simulink model "main_sim_adapt_Gref_SPPH"  (Simulink 7.2)
settings: Solver=ode2  SolverMode=SingleTasking  StartTime=0.0  StopTime=tsim_max  FixedStep=dtsim  RelTol=1e-3
StopFcn:
  | %mkplt
values from neighbouring files (symbols this model uses):
  assertion_time = inf    [setup_taem_sgs_al.m]
  cosA = cos(rwyAZ_rad)    [setup_taem_sgs_al.m]
  E_rwy = E_origin + (mod(( rwyLLA(2)/constants.r2d - lon_origin )+pi,2*pi)-pi) * constants.earth_radius * cos(lat_origin)    [setup_taem_sgs_al.m]
  eow_boundary = tmp_eow(ix(1))    [setup_taem_sgs_al.m]
  N_rwy = N_origin + (mod(( rwyLLA(1)/constants.r2d - lat_origin )+pi,2*pi)-pi) * constants.earth_radius    [setup_taem_sgs_al.m]
  sinA = sin(rwyAZ_rad)    [setup_taem_sgs_al.m]
  vel = 487.2512    [doit.m]
undefined symbols (not defined in the file or in its folder): accel_cmd, aero_surf_qbar_off, aero_surf_qbar_on, Alon, att_cmd_select, att_trim_IC, att_type, att_type_numbers, B1, bb_ellipsoid, bb_params, Blon, C, CA, chi_trim_IC, Clon, command_time, compute_all_rate_cols, compute_all_vel_cols, constants, da_trim_IC, dc_L2W_IC, de_trim_IC, DiscIntNeverNeededParam, dr_trim_IC, dtsim, DZkx, DZtheta, E_trim_IC, Ed_cmd, Ed_trim_IC, fc, flag_uad, full_surf_llim, full_surf_ulim, gain_set, gain_var_struct, gam_cmd_descent, gam_cmd_preflare, gamdot_cmd_descent, gamdot_cmd_flare, gamdot_cmd_preflare, gamma_trim_IC, Gamtheta, Gamx, h_trim_IC, hd_cmd, hd_trim_IC, ideal_vel_Kb, in_exsig_vecin, in_exsig_vecout, invCB, Kb, Kxhat0, Kxnom, Kxstar, lonxm0, MACH, MACH_att_fb, MACH_att_int_IC ... (+77)
libraries: simulink x36, utility_lib x36, mach_lib x24, model_lib x15, simulink_need_slupdate x8, models x6
(part 1 of 7)
CloseFcn:
  | rtwprivate ssgencode ModelCloseRequest main
settings Model: Creator=E183308  LastModifiedBy=E183308  ModifiedComment=E700252 -- Tue Nov 11 13:33:23 2003 -- Version 1.2477  TunableVars=MACH_U_nom_IC,MACH_gain_mat,MACH_mass_IC,MACH_pos_IC,MACH_pqr_Bmat_IC,MACH_pqr_u_IC,MACH_quat_IC,MACH_throttle_IC,MACH_vel_Bmat_IC,MACH_vel_IC,MACH_vel_cvdnom_IC,MACH_vel_uold_IC  TunableVarsStorageClass=Auto,Auto,Auto,Auto,Auto,Auto,Auto,Auto,Auto,Auto,Auto,Auto  TunableVarsTypeQualifier=,,,,,,,,,,,  BufferReuse=off
settings DataIOCC: LimitDataPoints=off  SaveOutput=off  SaveTime=off  SignalLoggingName=sigsOut
settings OptimizationCC: BlockReduction=off  BooleanDataType=off  BufferReuse=off  EnforceIntegerDowncast=off  FoldNonRolledExpr=off  InitFltsAndDblsToZero=on
settings DebuggingCC: SaveWithParameterizedLinksMsg=none  SignalResolutionControl=TryResolveAllWithWarning  SolverPrmCheckMsg=none  InheritedTsInSrcMsg=none  MultiTaskDSMMsg=warning  MultiTaskCondExecSysMsg=none  StrictBusMsg=ErrorLevel1
settings HardwareCC: TargetEndianess=LittleEndian  TargetHWDeviceType=MATLAB Host  ProdEqTarget=off
settings SFSimCC: SFSimEcho=off
settings RTWCC: SystemTargetFile=rtwsfcn.tlc  TemplateMakefile=rtwsfcn_default_tmf  Description=S-function Target  ProcessScript=rtwsfcn_make_rtw_hook  IncludeERTFirstTime=on
settings STFCustomTargetCC: TargetFcnLib=ansi_tfl_tmw.mat  ModelReferenceCompliant=off  SystemTargetFile=rtwsfcn.tlc
settings CustomProperty: Value=on

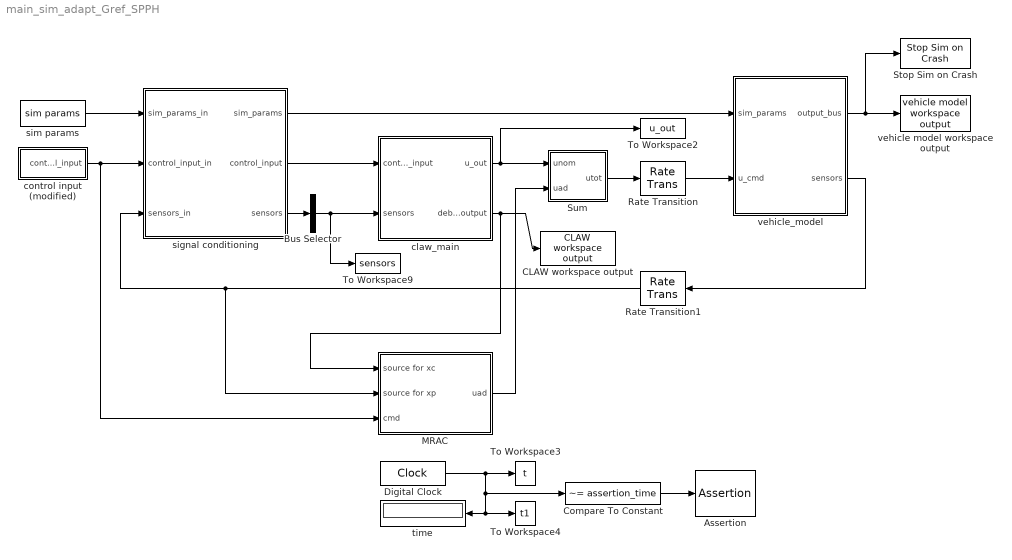
== system main_sim_adapt_Gref_SPPH ==
  Assertion : Assertion  Enabled=on  AssertionFailFcn=assertioncb  StopWhenAssertionFail=off
  Bus Selector : BusSelector  OutputSignals=pqr,NED_dot,latlonh,e,accels_cg,nav_ok,u_meas,NED_wind,seeker  OutputAsBus=on
  CLAW workspace output : mach_lib/CLAW workspace output  SystemSampleTime=-1
  Compare To Constant : simulink/Logic and Bit Operations/Compare To Constant  SystemSampleTime=-1  relop=~=  const=assertion_time  LogicOutDataTypeMode=boolean  ZeroCross=off
  Digital Clock : DigitalClock  SampleTime=dtsim
  MRAC : Subsystem  TreatAsAtomicUnit=on
  Rate Transition : RateTransition  X0=MACH_U_nom_IC
  Rate Transition1 : RateTransition  Orientation=left  OutPortSampleTime=MACH.dt
  Stop Sim on Crash : mach_lib/Stop Sim on Crash  SystemSampleTime=-1
  Sum : Subsystem
  To Workspace2 : ToWorkspace  VariableName=u_out  SampleTime=MACH.dt  SaveFormat=Array
  To Workspace3 : ToWorkspace  VariableName=t  SampleTime=dtsim  SaveFormat=Array
  To Workspace4 : ToWorkspace  VariableName=t1  SampleTime=MACH.dt  SaveFormat=Array
  To Workspace9 : ToWorkspace  VariableName=sensors  SampleTime=MACH.dt  SaveFormat=Array
      settings: MaxDataPoints=1
  claw_main : Subsystem  AncestorBlock=mach_lib/claw_main  TreatAsAtomicUnit=on  SystemSampleTime=MACH.dt
  control input (modified) : Subsystem
  signal conditioning : Subsystem
  sim params : mach_lib/sim params  SystemSampleTime=-1
  time : Display
  vehicle model workspace output : mach_lib/vehicle model workspace output  SystemSampleTime=-1
  vehicle_model : Subsystem  TreatAsAtomicUnit=on
  wires:
  Digital Clock/1 -> To Workspace3/1, Compare To Constant/1, time/1, To Workspace4/1
  claw_main/1(u_out) -> Sum/1(unom), To Workspace2/1
  vehicle_model/2(sensors) -> Rate Transition1/1
  claw_main/2(debug_output) -> CLAW workspace output/1, MRAC/1(source for xc)
  Rate Transition/1 -> vehicle_model/2(u_cmd)
  Bus Selector/1 -> To Workspace9/1, claw_main/2(sensors)
  vehicle_model/1(output_bus) -> vehicle model workspace output/1, Stop Sim on Crash/1
  Rate Transition1/1 -> signal conditioning/3(sensors_in), MRAC/2(source for xp)
  signal conditioning/3(sensors) -> Bus Selector/1
  signal conditioning/2(control_input) -> claw_main/1(control_input)
  sim params/1 -> signal conditioning/1(sim_params_in)
  signal conditioning/1(sim_params) -> vehicle_model/1(sim_params)
  Compare To Constant/1 -> Assertion/1
  MRAC/1(uad) -> Sum/2(uad)
  Sum/1(utot) -> Rate Transition/1
  control input (modified)/1(control_input) -> signal conditioning/2(control_input_in), MRAC/3(cmd)

== system main_sim_adapt_Gref_SPPH/MRAC ==
  source for xc : Inport
  source for xp : Inport  Port=2
  cmd : Inport  Port=3
  Adapt on (1.0 to 15 sec) : Subsystem  Tag=STV Subsys  LoadFcn=sigbuilder_block('load');  StartFcn=sigbuilder_block('start');  StopFcn=sigbuilder_block('stop');  ClipboardFcn=sigbuilder_block('clipboard');  mask(Sigbuilder block){}
      mask help: Sigbuilder GUI
      mask init:
      | if ~strcmp(get_param(bdroot(gcbh),'SimulationStatus'),'stopped') tuvar = sigbuilder_block('maskInit'); end
      settings: CopyFcn=sigbuilder_block('copy');  DeleteFcn=sigbuilder_block('delete');  ModelCloseFcn=sigbuilder_block('modelClose');  PreSaveFcn=sigbuilder_block('preSave');  NameChangeFcn=sigbuilder_block('namechange');  OpenFcn=sigbuilder_block('open',[223.5 120 685.5 399.75 ]);  CloseFcn=sigbuilder_block('close');
      mask Display: plot(0,0,100,100,[10,10,40,40,10],[80,20,20,80,80],[40,10],[50,50], [40,27,10],[65,72,56],[40,25,25,10],[28,28,43,43]);
  Bus Selector1 : BusSelector  OutputSignals=command  OutputAsBus=on
  Estimate of x : Subsystem
  MRAC Laws : Subsystem
  Ref Model (Short Period + Phugoid) : Subsystem
  Selector : Selector  InputPortWidth=4  IndexOptions=Index vector (dialog)  Indices=[2]  OutputSizes=1
  Sum : Sum  Inputs=-|+  OutDataType=sfix(16)  OutScaling=2^0
  Terminator : Terminator
  Terminator1 : Terminator
  To Workspace1 : ToWorkspace  VariableName=uad_xm  SampleTime=MACH.dt  SaveFormat=Array
  To Workspace2 : ToWorkspace  VariableName=uad_conv  SampleTime=MACH.dt  SaveFormat=Array
  To Workspace3 : ToWorkspace  VariableName=uad_x  SampleTime=MACH.dt  SaveFormat=Array
  command : Scope
      settings: YMin=0  YMax=15  SaveName=ScopeData6
  uad out : Scope
      settings: SaveName=ScopeData15
  uad : Outport  OutDataType=sfix(16)  OutScaling=2^0
  wires:
  Bus Selector1/1 -> Selector/1, MRAC Laws/3(r), command/1
  Selector/1 -> Ref Model (Short Period + Phugoid)/1(cmd)
  cmd/1 -> Bus Selector1/1
  MRAC Laws/1(uad) -> uad out/1, uad/1
  MRAC Laws/3(Kx_hat) -> Terminator/1
  MRAC Laws/4(Theta_hat) -> Terminator1/1
  source for xp/1 -> Estimate of x/2(In2)
  source for xc/1 -> Estimate of x/1(In1)
  Estimate of x/1(x) -> Sum/2, MRAC Laws/2(x), To Workspace3/1
  Sum/1 -> MRAC Laws/1(e)
  Adapt on (1.0 to 15 sec)/1(Signal 1) -> MRAC Laws/4(adapt on-off)
  MRAC Laws/2(uad_conv) -> To Workspace2/1
  Ref Model (Short Period + Phugoid)/1(xm) -> Sum/1, To Workspace1/1

== system main_sim_adapt_Gref_SPPH/Sum ==
  unom : Inport
  uad : Inport  Port=2
  Rate Transition1 : RateTransition  OutPortSampleTime=MACH.dt
  Sum : Sum  Inputs=|++  OutDataType=sfix(16)  OutScaling=2^0
  To Workspace1 : ToWorkspace  VariableName=elev_nom  SampleTime=MACH.dt  SaveFormat=Array
  To Workspace2 : ToWorkspace  VariableName=elev_adap  SampleTime=MACH.dt  SaveFormat=Array
  To Workspace9 : ToWorkspace  VariableName=elev_total  SampleTime=MACH.dt  SaveFormat=Array
  get RIE : Selector  InputPortWidth=MACH.num_u  IndexOptions=Index vector (dialog)  Indices=MACH.u_idx.elev  OutputSizes=1
  set RIE : Assignment  IndexOptions=Index vector (dialog)  Indices=MACH.u_idx.elev  OutputSizes=[1 1]
  utot : Outport
  wires:
  unom/1 -> get RIE/1, set RIE/1
  get RIE/1 -> Sum/1, To Workspace1/1
  uad/1 -> Rate Transition1/1
  Sum/1 -> set RIE/2, To Workspace9/1
  set RIE/1 -> utot/1
  Rate Transition1/1 -> To Workspace2/1, Sum/2

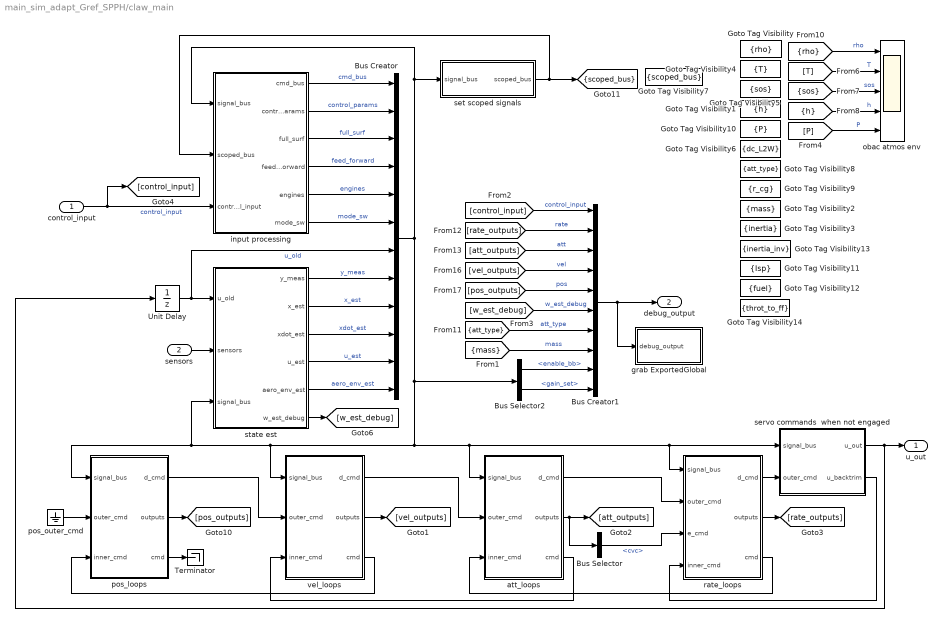
== system main_sim_adapt_Gref_SPPH/claw_main ==
  control_input : Inport  OutDataType=sfix(16)  OutScaling=2^0
      settings: BusObject=control_input_bus
  sensors : Inport  Port=2  OutDataType=sfix(16)  OutScaling=2^0
  Bus Creator : BusCreator  Inputs=12
  Bus Creator1 : BusCreator  Inputs=10
      settings: BusObject=CLAW_DEBUG_OUTPUT_BUS
  Bus Selector : BusSelector  OutputSignals=cvc
  Bus Selector2 : BusSelector  OutputSignals=control_params.enable_bb,control_params.gain_set
  Goto Tag Visibility : GotoTagVisibility  GotoTag=rho
  Goto Tag Visibility1 : GotoTagVisibility  GotoTag=h
  Goto Tag Visibility10 : GotoTagVisibility  GotoTag=P
  Goto Tag Visibility11 : GotoTagVisibility  GotoTag=Isp
  Goto Tag Visibility12 : GotoTagVisibility  GotoTag=fuel
  Goto Tag Visibility13 : GotoTagVisibility  GotoTag=inertia_inv
  Goto Tag Visibility14 : GotoTagVisibility  GotoTag=throt_to_ff
  Goto Tag Visibility2 : GotoTagVisibility  GotoTag=mass
  Goto Tag Visibility3 : GotoTagVisibility  GotoTag=inertia
  Goto Tag Visibility4 : GotoTagVisibility  GotoTag=T
  Goto Tag Visibility5 : GotoTagVisibility  GotoTag=sos
  Goto Tag Visibility6 : GotoTagVisibility  GotoTag=dc_L2W
  Goto Tag Visibility7 : GotoTagVisibility  GotoTag=scoped_bus
  Goto Tag Visibility8 : GotoTagVisibility  GotoTag=att_type
  Goto Tag Visibility9 : GotoTagVisibility  GotoTag=r_cg
  Terminator : Terminator
  Unit Delay : UnitDelay  X0=MACH_U_nom_IC  SampleTime=-1
  att_loops : Subsystem
  grab ExportedGlobal : Subsystem
  input processing : Subsystem
  obac atmos env : Scope  NumInputPorts=5
      settings: YMin=-5~-5~-5~-5~-5  YMax=5~5~5~5~5  SaveName=ScopeData2
  pos_loops : Subsystem
      settings: RTWSystemCode=Function
  pos_outer_cmd : Ground
  rate_loops : Subsystem
      settings: RTWSystemCode=Function
  servo commands  when not engaged : Subsystem
  set scoped signals : Subsystem
  state est : Subsystem
  vel_loops : Subsystem
      settings: RTWSystemCode=Function
  u_out : Outport  OutDataType=sfix(16)  OutScaling=2^0
  debug_output : Outport  Port=2  OutDataType=sfix(16)  OutScaling=2^0
  tag scope: scoped_bus=scoped
  wires:
  input processing/6(mode_sw) -> Bus Creator/6  "mode_sw"
  input processing/5(engines) -> Bus Creator/5  "engines"
  pos_loops/2(outputs) -> [pos_outputs]
  [pos_outputs] -> Bus Creator1/5  "pos"
  [vel_outputs] -> Bus Creator1/4  "vel"
  [att_outputs] -> Bus Creator1/3  "att"
  [rate_outputs] -> Bus Creator1/2  "rate"
  att_loops/1(d_cmd) -> rate_loops/2(outer_cmd)
  vel_loops/1(d_cmd) -> att_loops/2(outer_cmd)
  rate_loops/1(d_cmd) -> servo commands  when not engaged/2(outer_cmd)
  Bus Creator/1 -> att_loops/1(signal_bus), rate_loops/1(signal_bus), servo commands  when not engaged/1(signal_bus), vel_loops/1(signal_bus), pos_loops/1(signal_bus), state est/3(signal_bus), Bus Selector2/1, input processing/1(signal_bus), set scoped signals/1(signal_bus)
  pos_loops/3(cmd) -> Terminator/1
  att_loops/3(cmd) -> vel_loops/3(inner_cmd)
  rate_loops/3(cmd) -> att_loops/3(inner_cmd)
  pos_loops/1(d_cmd) -> vel_loops/2(outer_cmd)
  vel_loops/2(outputs) -> [vel_outputs]
  att_loops/2(outputs) -> [att_outputs], Bus Selector/1
  rate_loops/2(outputs) -> [rate_outputs]
  Bus Creator1/1 -> debug_output/1, grab ExportedGlobal/1(debug_output)
  Unit Delay/1 -> state est/1(u_old), Bus Creator/7  "u_old"
  sensors/1 -> state est/2(sensors)
  vel_loops/3(cmd) -> pos_loops/3(inner_cmd)
  servo commands  when not engaged/2(u_backtrim) -> rate_loops/4(inner_cmd)
  state est/4(u_est) -> Bus Creator/11  "u_est"
  state est/3(xdot_est) -> Bus Creator/10  "xdot_est"
  state est/2(x_est) -> Bus Creator/9  "x_est"
  state est/1(y_meas) -> Bus Creator/8  "y_meas"
  servo commands  when not engaged/1(u_out) -> u_out/1, Unit Delay/1
  pos_outer_cmd/1 -> pos_loops/2(outer_cmd)
  state est/6(w_est_debug) -> [w_est_debug]
  [w_est_debug] -> Bus Creator1/6  "w_est_debug"
  [att_type] -> Bus Creator1/7  "att_type"
  input processing/2(control_params) -> Bus Creator/2  "control_params"
  [h] -> obac atmos env/4  "h"
  [sos] -> obac atmos env/3  "sos"
  [T] -> obac atmos env/2  "T"
  [rho] -> obac atmos env/1  "rho"
  [P] -> obac atmos env/5  "P"
  state est/5(aero_env_est) -> Bus Creator/12  "aero_env_est"
  input processing/3(full_surf) -> Bus Creator/3  "full_surf"
  input processing/4(feed_forward) -> Bus Creator/4  "feed_forward"
  set scoped signals/1(scoped_bus) -> [scoped_bus], input processing/2(scoped_bus)
  [mass] -> Bus Creator1/8  "mass"
  Bus Selector2/1 -> Bus Creator1/9  "<enable_bb>"
  Bus Selector2/2 -> Bus Creator1/10  "<gain_set>"
  control_input/1 -> input processing/3(control_input), [control_input]  "control_input"
  input processing/1(cmd_bus) -> Bus Creator/1  "cmd_bus"
  [control_input] -> Bus Creator1/1  "control_input"
  Bus Selector/1 -> rate_loops/3(e_cmd)  "<cvc>"

== system main_sim_adapt_Gref_SPPH/control input (modified) ==
  Add Excitation : Subsystem
  Bus Assignment : BusAssignment  AssignedSignals=command
  control input : Subsystem  AncestorBlock=mach_lib/control input  SystemSampleTime=MACH.dt
  ideal responses : Subsystem  AncestorBlock=model_lib/ideal responses
  control_input : Outport
  wires:
  control input/1(control_input) -> Bus Assignment/1, Add Excitation/1(In)
  Add Excitation/1(Out) -> Bus Assignment/2
  Bus Assignment/1 -> control_input/1, ideal responses/1(control_input)

== system main_sim_adapt_Gref_SPPH/signal conditioning ==
  sim_params_in : Inport  OutDataType=sfix(16)  OutScaling=2^0
  control_input_in : Inport  Port=2  OutDataType=sfix(16)  OutScaling=2^0
  sensors_in : Inport  Port=3  OutDataType=sfix(16)  OutScaling=2^0
  Bus Assignment : BusAssignment  AssignedSignals=full_surf.full_surf_pref
  Bus Selector : BusSelector  OutputSignals=full_surf.full_surf_pref
  Compare To Constant : simulink/Logic and Bit Operations/Compare To Constant  SystemSampleTime=-1  relop=>=  const=0  LogicOutDataTypeMode=boolean  ZeroCross=off
  Compare To Constant1 : simulink/Logic and Bit Operations/Compare To Constant  SystemSampleTime=-1  relop=<=  const=5  LogicOutDataTypeMode=boolean  ZeroCross=off
  Constant : Constant  Value=360  OutDataType=sfix(16)  OutScaling=2^0
  Digital Clock : DigitalClock  SampleTime=MACH.dt
  Gain : Gain  Gain=0  ParameterDataType=sfix(16)  ParameterScaling=2^0  OutDataType=sfix(16)  OutScaling=2^0
  Logical Operator : Logic  AllPortsSameDT=off
  Product : Product  OutDataType=sfix(16)  OutScaling=2^0  RndMeth=Zero
  Sine Wave : Sin  TimeSource=Use external signal  Amplitude=5  Frequency=2*pi  SampleTime=0
  Sum : Sum  Inputs=|++  OutDataType=sfix(16)  OutScaling=2^0
  Sum1 : Sum  Inputs=|+-  OutDataType=sfix(16)  OutScaling=2^0
  get RIE : Selector  InputPortWidth=MACH.num_u  IndexOptions=Index vector (dialog)  Indices=MACH.vane_idx(1)  OutputSizes=1
  set RIE : Assignment  IndexOptions=Index vector (dialog)  Indices=MACH.vane_idx(1)  OutputSizes=[1 1]
  sim_params : Outport  OutDataType=sfix(16)  OutScaling=2^0
  control_input : Outport  Port=2  OutDataType=sfix(16)  OutScaling=2^0
  sensors : Outport  Port=3  OutDataType=sfix(16)  OutScaling=2^0
  wires:
  sim_params_in/1 -> sim_params/1
  control_input_in/1 -> Bus Assignment/1, Bus Selector/1
  sensors_in/1 -> sensors/1
  set RIE/1 -> Bus Assignment/2
  Sum/1 -> set RIE/2
  Bus Selector/1 -> set RIE/1, get RIE/1  "<full_surf_pref>"
  get RIE/1 -> Sum/1
  Digital Clock/1 -> Sum1/1
  Constant/1 -> Sum1/2
  Sum1/1 -> Sine Wave/1, Compare To Constant/1, Compare To Constant1/1
  Compare To Constant/1 -> Logical Operator/1
  Compare To Constant1/1 -> Logical Operator/2
  Logical Operator/1 -> Product/2
  Sine Wave/1 -> Product/1
  Product/1 -> Gain/1
  Bus Assignment/1 -> control_input/1
  Gain/1 -> Sum/2

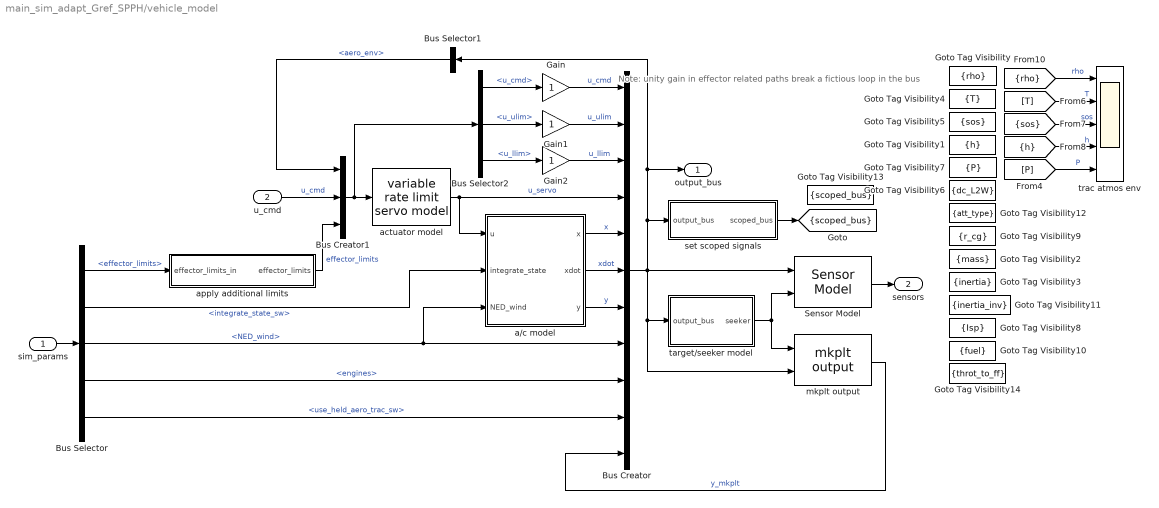
== system main_sim_adapt_Gref_SPPH/vehicle_model ==
  note: Note: unity gain in effector related paths
      | break a fictious loop in the bus
  sim_params : Inport  OutDataType=sfix(16)  OutScaling=2^0
  u_cmd : Inport  Port=2  OutDataType=sfix(16)  OutScaling=2^0
  Bus Creator : BusCreator  Inputs=11
  Bus Creator1 : BusCreator  Inputs=3
  Bus Selector : BusSelector  OutputSignals=effector_limits,integrate_state_sw,NED_wind,engines,use_held_aero_trac_sw
  Bus Selector1 : BusSelector  Orientation=left  OutputSignals=y.aero_env
  Bus Selector2 : BusSelector  OutputSignals=u_cmd,effector_limits.u_ulim,effector_limits.u_llim
  Gain : Gain  ParameterDataType=sfix(16)  ParameterScaling=2^0  OutDataType=sfix(16)  OutScaling=2^0
  Gain1 : Gain  ParameterDataType=sfix(16)  ParameterScaling=2^0  OutDataType=sfix(16)  OutScaling=2^0
  Gain2 : Gain  ParameterDataType=sfix(16)  ParameterScaling=2^0  OutDataType=sfix(16)  OutScaling=2^0
  Goto Tag Visibility : GotoTagVisibility  GotoTag=rho
  Goto Tag Visibility1 : GotoTagVisibility  GotoTag=h
  Goto Tag Visibility10 : GotoTagVisibility  GotoTag=fuel
  Goto Tag Visibility11 : GotoTagVisibility  GotoTag=inertia_inv
  Goto Tag Visibility12 : GotoTagVisibility  GotoTag=att_type
  Goto Tag Visibility13 : GotoTagVisibility  GotoTag=scoped_bus
  Goto Tag Visibility14 : GotoTagVisibility  GotoTag=throt_to_ff
  Goto Tag Visibility2 : GotoTagVisibility  GotoTag=mass
  Goto Tag Visibility3 : GotoTagVisibility  GotoTag=inertia
  Goto Tag Visibility4 : GotoTagVisibility  GotoTag=T
  Goto Tag Visibility5 : GotoTagVisibility  GotoTag=sos
  Goto Tag Visibility6 : GotoTagVisibility  GotoTag=dc_L2W
  Goto Tag Visibility7 : GotoTagVisibility  GotoTag=P
  Goto Tag Visibility8 : GotoTagVisibility  GotoTag=Isp
  Goto Tag Visibility9 : GotoTagVisibility  GotoTag=r_cg
  Sensor Model : model_lib/Sensor Model  SystemSampleTime=-1
  a/c model : Subsystem
  actuator model : model_lib/variable rate limit servo model  SystemSampleTime=-1
  apply additional limits : Subsystem
  mkplt output : model_lib/mkplt output  SystemSampleTime=-1
  set scoped signals : Subsystem
  target/seeker model : Subsystem
  trac atmos env : Scope  NumInputPorts=5
      settings: YMin=-5~-5~-5~-5~-5  YMax=5~5~5~5~5
  output_bus : Outport  OutDataType=sfix(16)  OutScaling=2^0
  sensors : Outport  Port=2  OutDataType=sfix(16)  OutScaling=2^0
  tag scope: scoped_bus=scoped
  wires:
  actuator model/1 -> a/c model/1(u), Bus Creator/4  "u_servo"
  Sensor Model/1 -> sensors/1
  Bus Selector/3 -> Bus Creator/8, a/c model/3(NED_wind)  "<NED_wind>"
  [h] -> trac atmos env/4  "h"
  [sos] -> trac atmos env/3  "sos"
  [T] -> trac atmos env/2  "T"
  [rho] -> trac atmos env/1  "rho"
  [P] -> trac atmos env/5  "P"
  target/seeker model/1(seeker) -> Sensor Model/2, mkplt output/1
  a/c model/1(x) -> Bus Creator/5  "x"
  a/c model/2(xdot) -> Bus Creator/6  "xdot"
  a/c model/3(y) -> Bus Creator/7  "y"
  Bus Creator/1 -> set scoped signals/1(output_bus), output_bus/1, Bus Selector1/1, target/seeker model/1(output_bus), mkplt output/2, Sensor Model/1
  sim_params/1 -> Bus Selector/1
  set scoped signals/1(scoped_bus) -> [scoped_bus]
  Bus Selector/4 -> Bus Creator/9  "<engines>"
  mkplt output/1 -> Bus Creator/11  "y_mkplt"
  Bus Selector/5 -> Bus Creator/10  "<use_held_aero_trac_sw>"
  Bus Creator1/1 -> actuator model/1, Bus Selector2/1
  Bus Selector1/1 -> Bus Creator1/1  "<aero_env>"
  u_cmd/1 -> Bus Creator1/2  "u_cmd"
  Bus Selector2/1 -> Gain/1  "<u_cmd>"
  Bus Selector2/2 -> Gain1/1  "<u_ulim>"
  Bus Selector2/3 -> Gain2/1  "<u_llim>"
  Gain/1 -> Bus Creator/1  "u_cmd"
  Gain1/1 -> Bus Creator/2  "u_ulim"
  Gain2/1 -> Bus Creator/3  "u_llim"
  Bus Selector/2 -> a/c model/2(integrate_state)  "<integrate_state_sw>"
  Bus Selector/1 -> apply additional limits/1(effector_limits_in)  "<effector_limits>"
  apply additional limits/1(effector_limits) -> Bus Creator1/3  "effector_limits"

== system main_sim_adapt_Gref_SPPH/MRAC/Adapt on (1.0 to 15 sec) ==
  Demux : Demux  Tag=STV Demux  Outputs=1
  FromWs : FromWorkspace  Tag=STV FromWs  VariableName=tuvar  SampleTime=0  SigBuilderData=DataTag0  VnvData=DataTag1
      SigBuilderData=|
      | common.afterFinalStr = 'Extrapolate'
      | common.sampleTime = 0
      | dataSet.timeRange = [0 25]
      | dataSet.name = 'Group 1'
      | sbobj.Groups.Signals.XData = [0 1 1 15 15 25]
      | sbobj.Groups.Signals.YData = [0 0 1 1 0 0]
  Signal 1 : Outport  Tag=STV Outport  OutDataType=sfix(16)  OutScaling=2^0
  wires:
  Demux/1 -> Signal 1/1
  FromWs/1 -> Demux/1

== system main_sim_adapt_Gref_SPPH/MRAC/Estimate of x ==
  In1 : Inport
  In2 : Inport  Port=2
  Bus Selector : BusSelector  OutputSignals=pqr,e,NED_dot,NED_wind
  Bus Selector22 : BusSelector  OutputSignals=rate.integ
  Constant1 : Constant  Orientation=left  Value=4.64*pi/180  OutDataType=sfix(16)  OutScaling=2^0
  Gain3 : Gain  Gain=180/pi  ParameterDataType=sfix(16)  ParameterScaling=2^0  OutDataType=sfix(16)  OutScaling=2^0
  Gain4 : Gain  Gain=180/pi  ParameterDataType=sfix(16)  ParameterScaling=2^0  OutDataType=sfix(16)  OutScaling=2^0
  Gain6 : Gain  Gain=180/pi  ParameterDataType=sfix(16)  ParameterScaling=2^0  OutDataType=sfix(16)  OutScaling=2^0
  K3 : Gain  Gain=-1/(fi*Kb)  ParameterDataType=sfix(16)  ParameterScaling=2^0  OutDataType=sfix(16)  OutScaling=2^0
  Mux : Mux  Inputs=3
  Product : Product  Multiplication=Matrix(*)  OutDataType=sfix(16)  OutScaling=2^0  SaturateOnIntegerOverflow=on  OutDataTypeStr=Inherit: Same as first input
  Reshape : Reshape  OutputDimensionality=Customize  OutputDimensions=[3,3]
  Selector1 : Selector  InputPortWidth=3  IndexOptions=Index vector (dialog)  Indices=[2]  OutputSizes=1
  Selector2 : Selector  InputPortWidth=3  IndexOptions=Index vector (dialog)  Indices=[2]  OutputSizes=1
  Sum1 : Sum  Inputs=|++  OutDataType=sfix(16)  OutScaling=2^0  SaturateOnIntegerOverflow=on
  Sum2 : Sum  Orientation=left  Inputs=|-+  OutDataType=sfix(16)  OutScaling=2^0
  Terminator2 : Terminator
  Terminator3 : Terminator
  alpha : Scope
      settings: YMin=-1  YMax=1  SaveName=ScopeData16
  del alpha : Scope
      settings: YMin=-1  YMax=1  SaveName=ScopeData25
  e2dc : utility_lib/e2dc  SystemSampleTime=-1
  q : Scope
      settings: SaveName=ScopeData11
  uvw_rw2Vab : utility_lib/uvw_rw2Vab  SystemSampleTime=-1
  xc : Scope
      settings: SaveName=ScopeData10
  x : Outport
  wires:
  Bus Selector/1 -> Selector1/1  "<pqr>"
  Bus Selector/2 -> e2dc/1  "<e>"
  Bus Selector22/1 -> Selector2/1  "<integ>"
  Selector2/1 -> K3/1
  e2dc/1 -> Reshape/1
  uvw_rw2Vab/2 -> Gain6/1, Sum2/2  "alpha"
  Gain6/1 -> alpha/1
  Sum1/1 -> Product/2
  Bus Selector/3 -> Sum1/1  "<NED_dot>"
  Bus Selector/4 -> Sum1/2  "<NED_wind>"
  Product/1 -> uvw_rw2Vab/1
  Reshape/1 -> Product/1
  uvw_rw2Vab/1 -> Terminator2/1
  uvw_rw2Vab/3 -> Terminator3/1
  Gain3/1 -> q/1
  Selector1/1 -> Gain3/1, Mux/2  "q"
  Sum2/1 -> Mux/3, Gain4/1
  Constant1/1 -> Sum2/1
  Gain4/1 -> del alpha/1
  In1/1 -> Bus Selector22/1
  Mux/1 -> x/1
  In2/1 -> Bus Selector/1
  K3/1 -> xc/1, Mux/1  "xc"

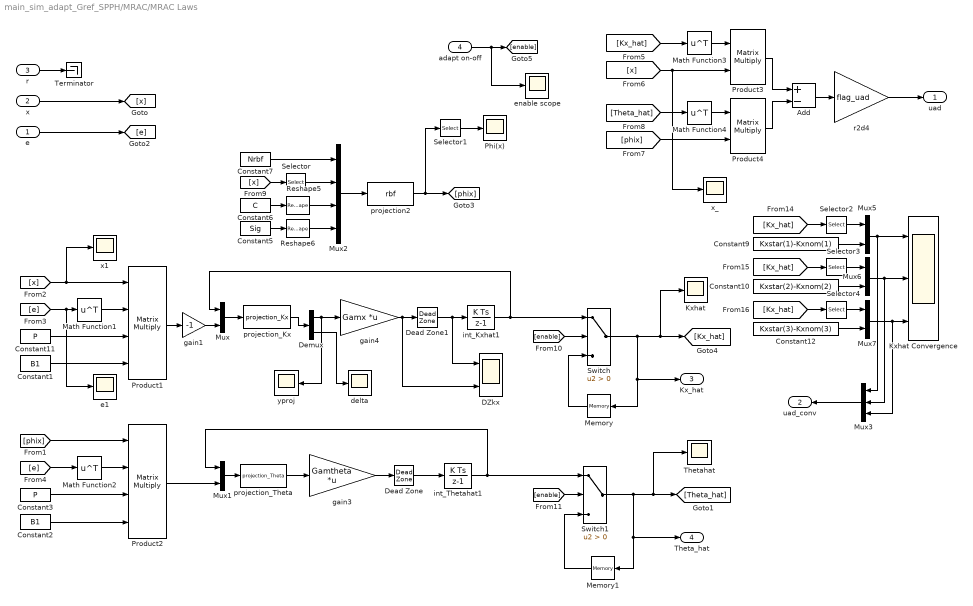
== system main_sim_adapt_Gref_SPPH/MRAC/MRAC Laws ==
  e : Inport  OutDataType=sfix(16)  OutScaling=2^0
  x : Inport  Port=2  OutDataType=sfix(16)  OutScaling=2^0
  r : Inport  Port=3  OutDataType=sfix(16)  OutScaling=2^0
  adapt on-off : Inport  Port=4  OutDataType=sfix(16)  OutScaling=2^0
  Add : Sum  Inputs=+-  OutDataType=sfix(16)  OutScaling=2^-10
  Constant1 : Constant  Value=B1  OutDataType=sfix(16)  OutScaling=2^0
  Constant10 : Constant  Value=Kxstar(2)-Kxnom(2)  OutDataType=sfix(16)  OutScaling=2^0
  Constant11 : Constant  Value=P  OutDataType=sfix(16)  OutScaling=2^0
  Constant12 : Constant  Value=Kxstar(3)-Kxnom(3)  OutDataType=sfix(16)  OutScaling=2^0
  Constant2 : Constant  Value=B1  OutDataType=sfix(16)  OutScaling=2^0
  Constant3 : Constant  Value=P  OutDataType=sfix(16)  OutScaling=2^0
  Constant5 : Constant  Value=Sig  OutDataType=sfix(16)  OutScaling=2^0
  Constant6 : Constant  Value=C  OutDataType=sfix(16)  OutScaling=2^0
  Constant7 : Constant  Value=Nrbf  OutDataType=sfix(16)  OutScaling=2^0
  Constant9 : Constant  Value=Kxstar(1)-Kxnom(1)  OutDataType=sfix(16)  OutScaling=2^0
  DZkx : Scope  NumInputPorts=2
      settings: TimeRange=20  YMin=-150~-150  YMax=250~250  SaveName=ScopeData14
  Dead Zone : DeadZone  LowerValue=-DZtheta  UpperValue=DZtheta  SaturateOnIntegerOverflow=on
  Dead Zone1 : DeadZone  LowerValue=-DZkx  UpperValue=DZkx  SaturateOnIntegerOverflow=on
  Demux : Demux  Outputs=[3 3]
  Kxhat : Scope
      settings: TimeRange=6  YMin=-2000  YMax=3500  SaveName=ScopeData4
  Kxhat Convergence : Scope  NumInputPorts=3
      settings: TimeRange=45  YMin=-50~-20~-50  YMax=150~140~200  SaveName=ScopeData13
  Math Function{1..4} (4 alike) : Math  Operator=transpose  OutDataType=sfix(16)  OutScaling=2^0  SaturateOnIntegerOverflow=on
  Memory : Memory  Orientation=left  X0=Kxhat0  InheritSampleTime=on
  Memory1 : Memory  Orientation=left  X0=Thetahat0  InheritSampleTime=on
  Mux : Mux  Inputs=2
  Mux1 : Mux  Inputs=2
  Mux2 : Mux
  Mux3 : Mux  Orientation=left  Inputs=3
  Mux5 : Mux  Inputs=[1 1]
  Mux6 : Mux  Inputs=[1 1]
  Mux7 : Mux  Inputs=[1 1]
  Phi(x) : Scope
      settings: TimeRange=40  YMin=-0.05  YMax=0.9  SaveName=ScopeData12
  Product1 : Product  Inputs=4  Multiplication=Matrix(*)  OutDataType=sfix(16)  OutScaling=2^0  RndMeth=Zero
  Product2 : Product  Inputs=4  Multiplication=Matrix(*)  OutDataType=sfix(16)  OutScaling=2^0  RndMeth=Zero
  Product3 : Product  Multiplication=Matrix(*)  OutDataType=sfix(16)  OutScaling=2^0  RndMeth=Zero
  Product4 : Product  Multiplication=Matrix(*)  OutDataType=sfix(16)  OutScaling=2^0  RndMeth=Zero
  Reshape5 : Reshape  OutputDimensions=[1,Nrbf]
  Reshape6 : Reshape  OutputDimensions=[Nrbf,1]
  Selector : Selector  InputPortWidth=nx  IndexOptions=Index vector (dialog)  Indices=3  OutputSizes=1
  Selector1 : Selector  InputPortWidth=11  IndexOptions=Select all  Indices=5  OutputSizes=1
  Selector2 : Selector  InputPortWidth=3  IndexOptions=Index vector (dialog)  Indices=1  OutputSizes=1
  Selector3 : Selector  InputPortWidth=3  IndexOptions=Index vector (dialog)  Indices=2  OutputSizes=1
  Selector4 : Selector  InputPortWidth=3  IndexOptions=Index vector (dialog)  Indices=3  OutputSizes=1
  Switch : Switch  Criteria=u2 > Threshold
  Switch1 : Switch  Criteria=u2 > Threshold
  Terminator : Terminator
  Thetahat : Scope
      settings: TimeRange=40  YMin=-0.3  YMax=0.4  SaveName=ScopeData7
  delta : Scope
      settings: TimeRange=40  YMin=-0.05  YMax=0.9
  e1 : Scope
      settings: TimeRange=25  YMin=-0.03  YMax=0.06  SaveName=ScopeData19
  enable scope : Scope
      settings: TimeRange=40  YMin=-0.05  YMax=0.9  SaveName=ScopeData17
  gain1 : Gain  Gain=-1  ParameterDataType=sfix(16)  ParameterScaling=2^0  OutDataType=sfix(16)  OutScaling=2^0
  gain3 : Gain  Gain=Gamtheta  Multiplication=Matrix(K*u)  ParameterDataType=sfix(16)  ParameterScaling=2^0  OutDataType=sfix(16)  OutScaling=2^0
  gain4 : Gain  Gain=Gamx  Multiplication=Matrix(K*u)  ParameterDataType=sfix(16)  ParameterScaling=2^0  OutDataType=sfix(16)  OutScaling=2^0
  int_Kxhat1 : DiscreteIntegrator  InitialCondition=Kxhat0  SampleTime=-1  OutDataType=sfix(16)  OutScaling=2^0  ICPrevOutput=DiscIntNeverNeededParam  ICPrevScaledInput=DiscIntNeverNeededParam
  int_Thetahat1 : DiscreteIntegrator  InitialCondition=Thetahat0  SampleTime=-1  OutDataType=sfix(16)  OutScaling=2^0  ICPrevOutput=DiscIntNeverNeededParam  ICPrevScaledInput=DiscIntNeverNeededParam
  projection2 : MATLABFcn  MATLABFcn=rbf  OutputDimensions=[Nrbf,1]  Output1D=off
  projection_Kx : MATLABFcn  MATLABFcn=projection_Kx
  projection_Theta : MATLABFcn  MATLABFcn=projection_Theta
  r2d4 : Gain  Gain=flag_uad  ParameterDataType=sfix(16)  ParameterScaling=2^0  OutDataType=sfix(16)  OutScaling=2^0
  x1 : Scope
      settings: TimeRange=40  YMin=-0.1  YMax=0.15  SaveName=ScopeData18
  x_ : Scope
      settings: TimeRange=40  YMin=-0.05  YMax=0.15  SaveName=ScopeData21
  yproj : Scope
      settings: TimeRange=25  YMin=-0.02  YMax=0.06  SaveName=ScopeData2
  uad : Outport  OutDataType=sfix(16)  OutScaling=2^0  InitialOutput=0
  uad_conv : Outport  Orientation=left  Port=2  OutDataType=sfix(16)  OutScaling=2^0  InitialOutput=0
  Kx_hat : Outport  Port=3  OutDataType=sfix(16)  OutScaling=2^0  InitialOutput=0
  Theta_hat : Outport  Port=4  OutDataType=sfix(16)  OutScaling=2^0  InitialOutput=0
  wires:
  Memory/1 -> Switch/3
  Memory1/1 -> Switch1/3
  adapt on-off/1 -> enable scope/1, [enable]
  [enable] -> Switch/2
  Switch/1 -> Memory/1, Kx_hat/1, Kxhat/1, [Kx_hat]
  [enable] -> Switch1/2
  Switch1/1 -> Memory1/1, Theta_hat/1, Thetahat/1, [Theta_hat]
  Demux/2 -> delta/1
  Demux/1 -> yproj/1, gain4/1
  projection_Kx/1 -> Demux/1
  gain4/1 -> DZkx/2, Dead Zone1/1
  Dead Zone1/1 -> DZkx/1, int_Kxhat1/1
  Mux7/1 -> Kxhat Convergence/3, Mux3/3
  Mux6/1 -> Kxhat Convergence/2, Mux3/2
  Mux5/1 -> Kxhat Convergence/1, Mux3/1
  Constant12/1 -> Mux7/2
  Selector4/1 -> Mux7/1
  [Kx_hat] -> Selector4/1
  Constant10/1 -> Mux6/2
  Selector3/1 -> Mux6/1
  [Kx_hat] -> Selector3/1
  Constant9/1 -> Mux5/2
  Selector2/1 -> Mux5/1
  [Kx_hat] -> Selector2/1
  Dead Zone/1 -> int_Thetahat1/1
  Selector1/1 -> Phi(x)/1
  r2d4/1 -> uad/1
  Selector/1 -> Mux2/2
  Reshape6/1 -> Mux2/4
  Reshape5/1 -> Mux2/3
  [x] -> Selector/1
  Constant7/1 -> Mux2/1
  projection2/1 -> Selector1/1, [phix]
  Mux2/1 -> projection2/1
  Constant5/1 -> Reshape6/1
  Constant6/1 -> Reshape5/1
  Add/1 -> r2d4/1
  Product4/1 -> Add/2
  Product3/1 -> Add/1
  [phix] -> Product4/2
  Math Function4/1 -> Product4/1
  [Theta_hat] -> Math Function4/1
  Mux1/1 -> projection_Theta/1
  gain3/1 -> Dead Zone/1
  projection_Theta/1 -> gain3/1
  Constant2/1 -> Product2/4
  Constant3/1 -> Product2/3
  Math Function2/1 -> Product2/2
  [phix] -> Product2/1
  Product2/1 -> Mux1/2
  [e] -> Math Function2/1
  Mux/1 -> projection_Kx/1
  gain1/1 -> Mux/2
  x/1 -> [x]
  Constant1/1 -> Product1/4
  Constant11/1 -> Product1/3
  Math Function1/1 -> Product1/2
  [x] -> x1/1, Product1/1
  Product1/1 -> gain1/1
  [x] -> Product3/2, x_/1
  Math Function3/1 -> Product3/1
  [Kx_hat] -> Math Function3/1
  [e] -> e1/1, Math Function1/1
  e/1 -> [e]
  r/1 -> Terminator/1
  int_Kxhat1/1 -> Switch/1, Mux/1
  int_Thetahat1/1 -> Switch1/1, Mux1/1
  Mux3/1 -> uad_conv/1

== system main_sim_adapt_Gref_SPPH/MRAC/Ref Model (Short Period + Phugoid) ==
  note: Desired
      | Dynamics
  note: Dynamic
      | Inversion
  note: OBAC
  cmd : Inport  OutDataType=sfix(16)  OutScaling=2^0
  Alon : Gain  Orientation=left  Gain=Alon  Multiplication=Matrix(K*u)  ParameterDataType=sfix(16)  ParameterScaling=2^0  OutDataType=sfix(16)  OutScaling=2^0
  Blon : Gain  Gain=Blon  Multiplication=Matrix(K*u)  ParameterDataType=sfix(16)  ParameterScaling=2^0  OutDataType=sfix(16)  OutScaling=2^0
  CA : Gain  Orientation=left  Gain=CA  Multiplication=Matrix(K*u)  ParameterDataType=sfix(16)  ParameterScaling=2^0  OutDataType=sfix(16)  OutScaling=2^0
  Clon : Gain  Gain=Clon  Multiplication=Matrix(K*u)  ParameterDataType=sfix(16)  ParameterScaling=2^0  OutDataType=sfix(16)  OutScaling=2^0
  Demux : Demux  Outputs=3
  Discrete-Time Integrator : DiscreteIntegrator  InitialCondition=lonxm0  SampleTime=-1  OutDataType=sfix(16)  OutScaling=2^0  ICPrevOutput=DiscIntNeverNeededParam  ICPrevScaledInput=DiscIntNeverNeededParam
  Discrete-Time Integrator1 : DiscreteIntegrator  SampleTime=-1  OutDataType=sfix(16)  OutScaling=2^0  ICPrevOutput=DiscIntNeverNeededParam  ICPrevScaledInput=DiscIntNeverNeededParam
  Gain : Gain  Gain=180/pi  ParameterDataType=sfix(16)  ParameterScaling=2^0  OutDataType=sfix(16)  OutScaling=2^0
  Gain1 : Gain  Gain=180/pi  ParameterDataType=sfix(16)  ParameterScaling=2^0  OutDataType=sfix(16)  OutScaling=2^0
  Gain2 : Gain  Gain=180/pi  ParameterDataType=sfix(16)  ParameterScaling=2^0  OutDataType=sfix(16)  OutScaling=2^0
  K : Gain  Gain=fi*Kb  ParameterDataType=sfix(16)  ParameterScaling=2^0  OutDataType=sfix(16)  OutScaling=2^0
  K1 : Gain  Gain=Kb  ParameterDataType=sfix(16)  ParameterScaling=2^0  OutDataType=sfix(16)  OutScaling=2^0
  K2 : Gain  Gain=fc  ParameterDataType=sfix(16)  ParameterScaling=2^0  OutDataType=sfix(16)  OutScaling=2^0
  K3 : Gain  Gain=-1/(fi*Kb)  ParameterDataType=sfix(16)  ParameterScaling=2^0  OutDataType=sfix(16)  OutScaling=2^0
  Mux : Mux  Inputs=[1 2]
  Sum1 : Sum  Inputs=|+-  OutDataType=sfix(16)  OutScaling=2^0
  Sum2 : Sum  Inputs=|++  OutDataType=sfix(16)  OutScaling=2^0
  Sum3 : Sum  Inputs=|+-  OutDataType=sfix(16)  OutScaling=2^0
  Sum4 : Sum  Inputs=++-  OutDataType=sfix(16)  OutScaling=2^0
  alpha (deg) : Scope
      settings: SaveName=ScopeData22
  invCB : Gain  Gain=invCB  Multiplication=Matrix(K*u)  ParameterDataType=sfix(16)  ParameterScaling=2^0  OutDataType=sfix(16)  OutScaling=2^0
  qcmd (deg/s) : Scope
      settings: YMin=-1  YMax=1  SaveName=ScopeData5
  qm (deg/s) : Scope
      settings: SaveName=ScopeData3
  qm2 : Selector  Orientation=left  InputPortWidth=2  IndexOptions=Index vector (dialog)  Indices=1  OutputSizes=1
  xcm : Scope
      settings: SaveName=ScopeData9
  xm : Outport  OutDataType=sfix(16)  OutScaling=2^0
  wires:
  Demux/1 -> xcm/1
  Gain2/1 -> qcmd (deg/s)/1
  Gain1/1 -> alpha (deg)/1
  Gain/1 -> qm (deg/s)/1
  Demux/3 -> Gain1/1
  Demux/2 -> Gain/1
  Blon/1 -> Sum2/1
  Sum2/1 -> Discrete-Time Integrator/1
  Alon/1 -> Sum2/2
  Discrete-Time Integrator/1 -> Alon/1, Clon/1  "xc"
  Clon/1 -> Mux/2, CA/1, qm2/1  "xp = [q alpha]'"
  CA/1 -> Sum1/2
  Sum1/1 -> invCB/1
  invCB/1 -> Blon/1
  cmd/1 -> Sum3/1, K2/1, Gain2/1
  K/1 -> Discrete-Time Integrator1/1
  Sum3/1 -> K/1
  Discrete-Time Integrator1/1 -> Sum4/2, K3/1  "xc"
  Sum4/1 -> K1/1
  K2/1 -> Sum4/1
  K1/1 -> Sum1/1
  qm2/1 -> Sum4/3, Sum3/2
  Mux/1 -> xm/1, Demux/1
  K3/1 -> Mux/1

== system main_sim_adapt_Gref_SPPH/claw_main/att_loops ==
  signal_bus : Inport  OutDataType=sfix(16)  OutScaling=2^0
  outer_cmd : Inport  Port=2  OutDataType=sfix(16)  OutScaling=2^0
  inner_cmd : Inport  Port=3  OutDataType=sfix(16)  OutScaling=2^0
  Bus Creator : BusCreator  Inputs=7
  Bus Selector : BusSelector  OutputSignals=control_params.limit_pqr_cmd,x_est.uvw,x_est.e
  Bus Selector4 : BusSelector  OutputSignals=feed_forward.att_ff,mode_sw.int_reset_sw,control_params.att_desdyn
  Demux1 : Demux  Outputs=[ MACH.att_num_u MACH.num_u_throt ]
  Mux2 : Mux  Inputs=2
  P+I+AW+TRIM Control : Subsystem
  compute trim : Subsystem
  dc2mba : utility_lib/dc2mba  SystemSampleTime=-1
  dc2tiltcam : utility_lib/dc2tiltcam  SystemSampleTime=-1
  dc2ypr : utility_lib/dc2ypr  SystemSampleTime=-1
  dyn inv : Subsystem
  e2dc : utility_lib/e2dc  SystemSampleTime=-1
  low pass filter : Subsystem
  select att cmd : Subsystem
  d_cmd : Outport  OutDataType=sfix(16)  OutScaling=2^0
  outputs : Outport  Port=2  OutDataType=sfix(16)  OutScaling=2^0
  cmd : Outport  Port=3  OutDataType=sfix(16)  OutScaling=2^0
  wires:
  Mux2/1 -> d_cmd/1
  [throt] -> Mux2/2
  P+I+AW+TRIM Control/2(int state) -> Bus Creator/2  "integ"
  dyn inv/3(cvdex) -> [cvdex], Bus Creator/1  "cvdex"
  Bus Selector/3 -> select att cmd/1(e_current), dyn inv/3(e nom), [cv], P+I+AW+TRIM Control/1(cv)  "<e>"
  outer_cmd/1 -> select att cmd/3(outer cmd)
  P+I+AW+TRIM Control/1(cvdot des) -> dyn inv/4(e dot des)
  [cvdex] -> P+I+AW+TRIM Control/4(cvdot extra)
  dyn inv/1(Bmat) -> compute trim/2(Bmat)
  [trim] -> P+I+AW+TRIM Control/5(trim)
  signal_bus/1 -> Bus Selector/1, select att cmd/4(signal_bus), Bus Selector4/1, low pass filter/2(signal_bus)
  compute trim/1(trim) -> [trim]
  select att cmd/2(throt_cmd) -> [throt]
  [cvc] -> Bus Creator/3, e2dc/1  "cvc"
  Bus Creator/1 -> outputs/1
  inner_cmd/1 -> Demux1/1
  Demux1/1 -> compute trim/1(inner cmd)
  Demux1/2 -> [throt_inner]
  dc2tiltcam/1 -> Bus Creator/5  "tiltcam_cmds"
  [cv] -> Bus Creator/4  "cv"
  e2dc/1 -> dc2tiltcam/1, dc2ypr/1, dc2mba/1
  dc2ypr/1 -> Bus Creator/6  "rpy_cmds"
  dc2mba/1 -> Bus Creator/7  "mab_cmds"
  Bus Selector/2 -> dyn inv/2(uvw)  "<uvw>"
  Bus Selector4/3 -> P+I+AW+TRIM Control/7(x0)  "<att_desdyn>"
  select att cmd/3(cmd) -> cmd/1
  dyn inv/2(pqr) -> Mux2/1, compute trim/3(cmd)
  Bus Selector4/2 -> P+I+AW+TRIM Control/6(reset)  "<int_reset_sw>"
  Bus Selector/1 -> dyn inv/1(limit_pqr_cmd)  "<limit_pqr_cmd>"
  [throt_inner] -> select att cmd/2(throt_current)
  select att cmd/1(e_cmd) -> low pass filter/1(e_cmd), [cvc]
  low pass filter/1(cv cmd) -> P+I+AW+TRIM Control/2(cv cmd)
  low pass filter/2(cvd ff) -> P+I+AW+TRIM Control/3(cvd ff)
  Bus Selector4/1 -> low pass filter/3(att_ff)  "<att_ff>"

== system main_sim_adapt_Gref_SPPH/claw_main/grab ExportedGlobal ==
  debug_output : Inport  OutDataType=sfix(16)  OutScaling=2^0
  Terminator{1..4,6} (5 alike) : Terminator
  grab cv variables : Subsystem
  grab cvcmd variables : Subsystem
  grab cvdex variables : Subsystem
  grab integrator variables : Subsystem
  grab w_est variables : Subsystem
  wires:
  debug_output/1 -> grab cv variables/1(In1), grab w_est variables/1(In1), grab cvcmd variables/1(In1), grab integrator variables/1(In1), grab cvdex variables/1(In1)
  grab cvdex variables/1(Out1) -> Terminator1/1
  grab integrator variables/1(Out1) -> Terminator2/1
  grab cvcmd variables/1(Out1) -> Terminator3/1
  grab cv variables/1(Out1) -> Terminator4/1
  grab w_est variables/1(Out1) -> Terminator6/1

== system main_sim_adapt_Gref_SPPH/claw_main/input processing ==
  signal_bus : Inport  OutDataType=sfix(16)  OutScaling=2^0
  scoped_bus : Inport  Port=2  OutDataType=sfix(16)  OutScaling=2^0
  control_input : Inport  Port=3  OutDataType=sfix(16)  OutScaling=2^0
  Bus Selector2 : BusSelector  OutputSignals=full_surf
  Bus Selector3 : BusSelector  OutputSignals=engines,mode_sw,command
  Bus Selector4 : BusSelector  OutputSignals=u_old,y_meas.u_meas
  mode dependent stick processing : Subsystem
  modify limits and apply to direct commands : Subsystem
  select att_type : Subsystem
  set control parameters : Subsystem
  cmd_bus : Outport  OutDataType=sfix(16)  OutScaling=2^0
  control_params : Outport  Port=2  OutDataType=sfix(16)  OutScaling=2^0
  full_surf : Outport  Port=3  OutDataType=sfix(16)  OutScaling=2^0
  feed_forward : Outport  Port=4  OutDataType=sfix(16)  OutScaling=2^0
  engines : Outport  Port=5  OutDataType=sfix(16)  OutScaling=2^0
  mode_sw : Outport  Port=6  OutDataType=sfix(16)  OutScaling=2^0
  wires:
  Bus Selector3/1 -> engines/1  "<engines>"
  mode dependent stick processing/1(cmd_bus) -> cmd_bus/1
  Bus Selector3/3 -> mode dependent stick processing/1(command)  "<command>"
  set control parameters/1(control_params) -> control_params/1
  Bus Selector4/1 -> modify limits and apply to direct commands/1(u_old)  "<u_old>"
  Bus Selector2/1 -> modify limits and apply to direct commands/3(full_surf_in)  "<full_surf>"
  modify limits and apply to direct commands/1(full_surf) -> full_surf/1, set control parameters/2(full_surf)
  control_input/1 -> Bus Selector3/1, Bus Selector2/1
  signal_bus/1 -> set control parameters/1(signal_bus), Bus Selector4/1, mode dependent stick processing/2(signal_bus), select att_type/3(signal_bus)
  mode dependent stick processing/2(feed_forward) -> feed_forward/1
  Bus Selector3/2 -> select att_type/2(mode_sw_in)  "<mode_sw>"
  scoped_bus/1 -> select att_type/1(scoped_bus)
  select att_type/1(mode_sw) -> mode_sw/1
  Bus Selector4/2 -> modify limits and apply to direct commands/2(u_meas)  "<u_meas>"

== system main_sim_adapt_Gref_SPPH/claw_main/pos_loops ==
  signal_bus : Inport  OutDataType=sfix(16)  OutScaling=2^0
  outer_cmd : Inport  Port=2  OutDataType=sfix(16)  OutScaling=2^0
  inner_cmd : Inport  Port=3  OutDataType=sfix(16)  OutScaling=2^0
  Bus Creator : BusCreator  Inputs=5
  Bus Selector : BusSelector  OutputSignals=feed_forward.pos_ff,mode_sw.int_reset_sw,control_params.pos_desdyn,y_meas.dc_fltpath
  Bus Selector1 : BusSelector  OutputSignals=x_est.NEh
  Mux : Mux  Inputs=[3 1 ]
  P+I+AW+TRIM Control : mach_lib/P+I+AW+TRIM Control  SystemSampleTime=-1
  Product : Product  Multiplication=Matrix(*)  OutDataType=sfix(16)  OutScaling=2^0  RndMeth=Zero
  Selector1 : Selector  InputPortWidth=4  IndexOptions=Index vector (dialog)  Indices=[1 2 4]  OutputSizes=1
  Selector3 : Selector  InputPortWidth=4  IndexOptions=Index vector (dialog)  Indices=[1 2 4 3]  OutputSizes=1
  compute trim : Subsystem
  limiter : Subsystem
  select pos cmd : Subsystem
  d_cmd : Outport  OutDataType=sfix(16)  OutScaling=2^0
  outputs : Outport  Port=2  OutDataType=sfix(16)  OutScaling=2^0
  cmd : Outport  Port=3  OutDataType=sfix(16)  OutScaling=2^0
  wires:
  [camcmd] -> Mux/2
  Mux/1 -> Selector3/1
  select pos cmd/1(NEh_cmd) -> P+I+AW+TRIM Control/2, [cvc]
  Bus Selector1/1 -> P+I+AW+TRIM Control/1, [cv], select pos cmd/1(NEh_current)  "<NEh>"
  signal_bus/1 -> Bus Selector/1, select pos cmd/3(signal_bus), Bus Selector1/1, limiter/2(signal_bus)
  compute trim/1(trim) -> [trim]
  inner_cmd/1 -> Selector1/1
  Selector1/1 -> compute trim/1(inner cmd), limiter/1(vel_inner_cmd)
  outer_cmd/1 -> select pos cmd/2(outer cmd)
  select pos cmd/3(cmd) -> cmd/1
  Selector3/1 -> d_cmd/1
  [cvc] -> Bus Creator/3  "cvc"
  [cv] -> Bus Creator/4  "cv"
  [trim] -> P+I+AW+TRIM Control/5
  [cvdex] -> P+I+AW+TRIM Control/4
  Bus Selector/2 -> P+I+AW+TRIM Control/6  "<int_reset_sw>"
  Bus Selector/3 -> P+I+AW+TRIM Control/7  "<pos_desdyn>"
  limiter/1(cvd_des) -> Mux/1, compute trim/2(cmd)
  P+I+AW+TRIM Control/1 -> limiter/3(cvd_des_in)
  [cvdex] -> Product/2
  P+I+AW+TRIM Control/2 -> Bus Creator/2  "integ"
  Bus Creator/1 -> outputs/1
  Bus Selector/4 -> Product/1  "<dc_fltpath>"
  Product/1 -> Bus Creator/5  "cvdex_fltpath"
  limiter/2(cvd_extra) -> Bus Creator/1, [cvdex]  "cvdex"
  Bus Selector/1 -> P+I+AW+TRIM Control/3  "<pos_ff>"
  select pos cmd/2(cam_cmd) -> [camcmd]

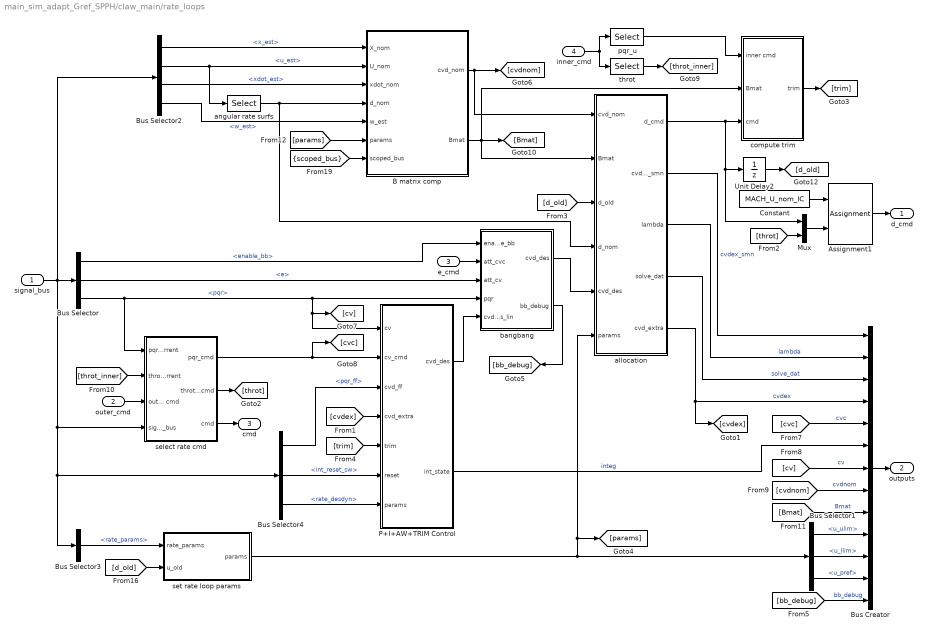
== system main_sim_adapt_Gref_SPPH/claw_main/rate_loops ==
  signal_bus : Inport  OutDataType=sfix(16)  OutScaling=2^0
  outer_cmd : Inport  Port=2  OutDataType=sfix(16)  OutScaling=2^0
  e_cmd : Inport  Port=3  OutDataType=sfix(16)  OutScaling=2^0
  inner_cmd : Inport  Port=4  OutDataType=sfix(16)  OutScaling=2^0
  Assignment1 : Assignment  IndexOptions=Index vector (dialog)  Indices=[MACH.pqr_u_idx MACH.throttle_idx]  OutputSizes=[1 1]
  B matrix comp : Subsystem  TreatAsAtomicUnit=on
  Bus Creator : BusCreator  Inputs=13
  Bus Selector : BusSelector  OutputSignals=control_params.enable_bb,x_est.e,x_est.pqr
  Bus Selector1 : BusSelector  OutputSignals=u_ulim,u_llim,u_pref
  Bus Selector2 : BusSelector  OutputSignals=x_est,u_est,xdot_est,y_meas.w_est
  Bus Selector3 : BusSelector  OutputSignals=control_params.rate_params
  Bus Selector4 : BusSelector  OutputSignals=feed_forward.pqr_ff,mode_sw.int_reset_sw,control_params.rate_desdyn
  Constant : Constant  Value=MACH_U_nom_IC  OutDataType=sfix(16)  OutScaling=2^0
  Mux : Mux  Inputs=2
  P+I+AW+TRIM Control : Subsystem  AncestorBlock=mach_lib/P+I+AW+TRIM Control
  Unit Delay2 : UnitDelay  X0=MACH_pqr_u_IC  SampleTime=-1
  allocation : Subsystem
  angular rate surfs : Selector  InputPortWidth=MACH.num_u  IndexOptions=Index vector (dialog)  Indices=MACH.pqr_u_idx  OutputSizes=1
  bangbang : Subsystem
  compute trim : Subsystem
  pqr_u : Selector  InputPortWidth=MACH.num_u  IndexOptions=Index vector (dialog)  Indices=MACH.pqr_u_idx  OutputSizes=1
  select rate cmd : Subsystem
  set rate loop params : Subsystem
  throt : Selector  InputPortWidth=MACH.num_u  IndexOptions=Index vector (dialog)  Indices=MACH.throttle_idx  OutputSizes=1
  d_cmd : Outport  OutDataType=sfix(16)  OutScaling=2^0
  outputs : Outport  Port=2  OutDataType=sfix(16)  OutScaling=2^0
  cmd : Outport  Port=3  OutDataType=sfix(16)  OutScaling=2^0
  wires:
  angular rate surfs/1 -> B matrix comp/4(d_nom), allocation/4(d_nom)
  outer_cmd/1 -> select rate cmd/3(outer cmd)
  B matrix comp/1(cvd_nom) -> [cvdnom], allocation/1(cvd_nom)
  P+I+AW+TRIM Control/2(int_state) -> Bus Creator/6  "integ"
  signal_bus/1 -> Bus Selector2/1, Bus Selector/1, Bus Selector3/1, Bus Selector4/1, select rate cmd/4(signal_bus)
  compute trim/1(trim) -> [trim]
  inner_cmd/1 -> pqr_u/1, throt/1
  select rate cmd/2(throt_cmd) -> [throt]
  select rate cmd/1(pqr_cmd) -> [cvc], P+I+AW+TRIM Control/2(cv_cmd)
  [throt_inner] -> select rate cmd/2(throt_current)
  [cvc] -> Bus Creator/5  "cvc"
  [cv] -> Bus Creator/7  "cv"
  [cvdnom] -> Bus Creator/8  "cvdnom"
  set rate loop params/1(params) -> Bus Selector1/1, allocation/6(params), [params]
  Assignment1/1 -> d_cmd/1
  throt/1 -> [throt_inner]
  [trim] -> P+I+AW+TRIM Control/5(trim)
  [cvdex] -> P+I+AW+TRIM Control/4(cvd_extra)
  Bus Selector/3 -> select rate cmd/1(pqr_current), bangbang/4(pqr), P+I+AW+TRIM Control/1(cv), [cv]  "<pqr>"
  Bus Selector4/1 -> P+I+AW+TRIM Control/3(cvd_ff)  "<pqr_ff>"
  Bus Selector4/2 -> P+I+AW+TRIM Control/6(reset)  "<int_reset_sw>"
  [Bmat] -> Bus Creator/9  "Bmat"
  Bus Selector1/1 -> Bus Creator/10  "<u_ulim>"
  Bus Selector1/2 -> Bus Creator/11  "<u_llim>"
  [d_old] -> set rate loop params/2(u_old)
  pqr_u/1 -> compute trim/1(inner cmd)
  Constant/1 -> Assignment1/1
  Mux/1 -> Assignment1/2
  Bus Selector2/1 -> B matrix comp/1(X_nom)  "<x_est>"
  Bus Selector2/2 -> angular rate surfs/1, B matrix comp/2(U_nom)  "<u_est>"
  Bus Selector2/3 -> B matrix comp/3(xdot_nom)  "<xdot_est>"
  Bus Selector2/4 -> B matrix comp/5(w_est)  "<w_est>"
  Bus Selector1/3 -> Bus Creator/12  "<u_pref>"
  allocation/5(cvd_extra) -> Bus Creator/4, [cvdex]  "cvdex"
  [throt] -> Mux/2
  Unit Delay2/1 -> [d_old]
  allocation/1(d_cmd) -> compute trim/3(cmd), Mux/1, Unit Delay2/1
  [d_old] -> allocation/3(d_old)
  B matrix comp/2(Bmat) -> compute trim/2(Bmat), [Bmat], allocation/2(Bmat)
  allocation/3(lambda) -> Bus Creator/2  "lambda"
  allocation/4(solve_dat) -> Bus Creator/3  "solve_dat"
  Bus Creator/1 -> outputs/1
  [scoped_bus] -> B matrix comp/7(scoped_bus)
  [params] -> B matrix comp/6(params)
  Bus Selector4/3 -> P+I+AW+TRIM Control/7(params)  "<rate_desdyn>"
  allocation/2(cvd_extra_smn) -> Bus Creator/1  "cvdex_smn"
  bangbang/1(cvd_des) -> allocation/5(cvd_des)
  e_cmd/1 -> bangbang/2(att_cvc)
  Bus Selector/2 -> bangbang/3(att_cv)  "<e>"
  P+I+AW+TRIM Control/1(cvd_des) -> bangbang/5(cvd_des_lin)
  Bus Selector/1 -> bangbang/1(enable_bb)  "<enable_bb>"
  bangbang/2(bb_debug) -> [bb_debug]
  [bb_debug] -> Bus Creator/13  "bb_debug"
  select rate cmd/3(cmd) -> cmd/1
  Bus Selector3/1 -> set rate loop params/1(rate_params)  "<rate_params>"

== system main_sim_adapt_Gref_SPPH/claw_main/servo commands  when not engaged ==
  note: for OAV/MAV during "pre-takeoff",
      |  the rate inner_cmd throt was set to takeoff throt
      | to allow integrators to trim for anticipated takeoff.
      | This should be revisited within current CLAW
      | before being used again.
  signal_bus : Inport  OutDataType=sfix(16)  OutScaling=2^0
  outer_cmd : Inport  Port=2  OutDataType=sfix(16)  OutScaling=2^0
  Bus Selector1 : BusSelector  OutputSignals=mode_sw.pre_takeoff_sw,mode_sw.engaged_sw,mode_sw.full_surf_cmd_sw,cmd_bus.autopilot_cmd,full_surf.full_surf_cmd
  Constant1 : Constant  Value=MACH.pre_takeoff_u_backtrim  OutDataType=sfix(16)  OutScaling=2^0
  Multiport Switch : MultiPortSwitch  Inputs=2  zeroidx=on
  Multiport Switch1 : MultiPortSwitch  Inputs=2  zeroidx=on
  Multiport Switch2 : MultiPortSwitch  Inputs=2  zeroidx=on
  pseudo surf cmd : Subsystem
  u_out : Outport  OutDataType=sfix(16)  OutScaling=2^0
  u_backtrim : Outport  Port=2  OutDataType=sfix(16)  OutScaling=2^0
  wires:
  signal_bus/1 -> Bus Selector1/1
  Bus Selector1/1 -> Multiport Switch/1  "<pre_takeoff_sw>"
  Multiport Switch1/1 -> Multiport Switch/2, u_out/1
  Constant1/1 -> Multiport Switch/3
  Bus Selector1/2 -> Multiport Switch1/1  "<engaged_sw>"
  Bus Selector1/3 -> Multiport Switch2/1  "<full_surf_cmd_sw>"
  Bus Selector1/4 -> pseudo surf cmd/1(autopilot_cmd)  "<autopilot_cmd>"
  pseudo surf cmd/1(surf_cmd) -> Multiport Switch2/2
  Bus Selector1/5 -> Multiport Switch2/3  "<full_surf_cmd>"
  Multiport Switch2/1 -> Multiport Switch1/2
  outer_cmd/1 -> Multiport Switch1/3
  Multiport Switch/1 -> u_backtrim/1
